simulink model "q3fullcontrolledSON"  (R2018a)
settings: Solver=VariableStepAuto  StartTime=0.0  StopTime=2  RelTol=1e-6
libraries: powerlib x14, powerlib_meascontrol x2
settings Model: Creator=asus  LastModifiedBy=asus

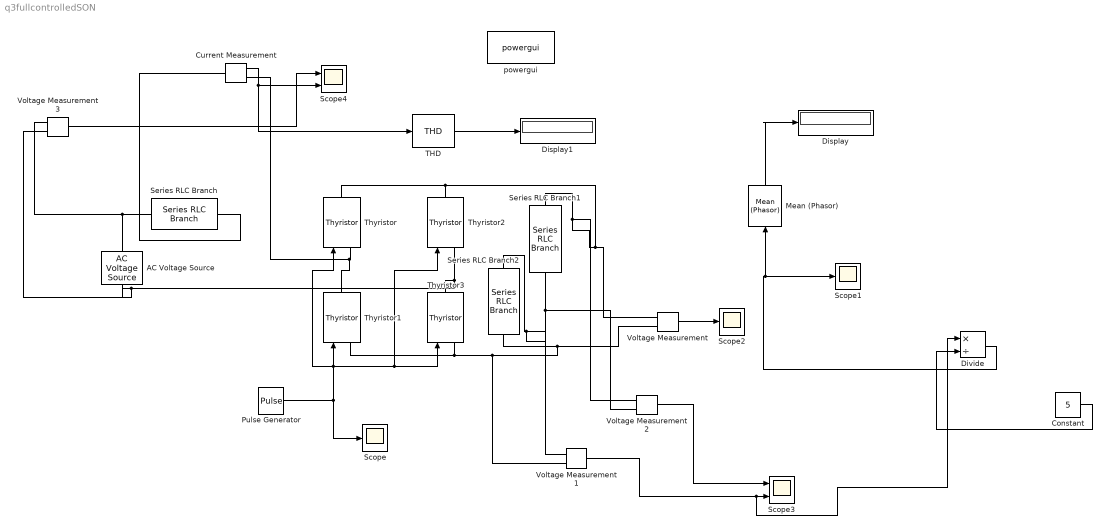
== system q3fullcontrolledSON ==
  AC Voltage Source : powerlib/Electrical Sources/AC Voltage Source  Amplitude=325.2  Phase=0  Frequency=50  SampleTime=0  Measurements=None  BusType=swing  Pref=10e3  Qref=0  Qmin=-inf  Qmax=+inf
  Constant : Constant  Value=5
  Current Measurement : powerlib/Measurements/Current Measurement  PhasorSimulation=off  OutputType=Complex  PSBequivalent=0
  Display : Display
  Display1 : Display
  Divide : Product  Inputs=*/
  Mean (Phasor) : powerlib_meascontrol/Measurements/Mean (Phasor)  Freq=60  Vinit=0  Ts=0
      settings: SourceProductName=Simscape Power Systems  SourceProductBaseCode=PS
  Pulse Generator : DiscretePulseGenerator  PulseType=Time based  Amplitude=10  Period=1e-2  PulseWidth=5  PhaseDelay=2.41e-3
  Scope : Scope
  Scope1 : Scope
  Scope2 : Scope
  Scope3 : Scope  NumInputPorts=2
  Scope4 : Scope  NumInputPorts=2
  Series RLC Branch : powerlib/Elements/Series RLC Branch  LConnTagsString=__new0  RConnTagsString=__new0  BranchType=L  Resistance=1  Inductance=5e-4  SetiL0=off  InitialCurrent=0  Capacitance=1e-6  Setx0=off  InitialVoltage=0  Measurements=None
  Series RLC Branch1 : powerlib/Elements/Series RLC Branch  LConnTagsString=__new0  RConnTagsString=__new0  BranchType=L  Resistance=1  Inductance=250e-3  SetiL0=off  InitialCurrent=0  Capacitance=1e-6  Setx0=off  InitialVoltage=0  Measurements=None
  Series RLC Branch2 : powerlib/Elements/Series RLC Branch  LConnTagsString=__new0  RConnTagsString=__new0  BranchType=R  Resistance=5  Inductance=1e-3  SetiL0=off  InitialCurrent=0  Capacitance=1e-6  Setx0=off  InitialVoltage=0  Measurements=None
  THD : powerlib_meascontrol/Measurements/THD  Freq=60  Ts=0
  Thyristor{,1..3} (4 alike) : powerlib/Power Electronics/Thyristor  Ron=1e-9  Lon=0  Vf=0  IC=0  Rs=500  Cs=1e-9  Measurements=off
  Voltage Measurement{,1..3} (4 alike) : powerlib/Measurements/Voltage Measurement  PhasorSimulation=off  OutputType=Complex  PSBequivalent=0
  powergui : powerlib/powergui  Priority=1  SimulationMode=Discrete  SampleTime=5e-6  frequency=60  Iterations=50  frequencyindice=50  Pbase=100e6  ErrMax=1e-4  UnitsV=kV  UnitsW=MW  buscounter=0  FunctionMessages=off  echomessages=off  EnableUseOfTLC=off  CurrentSourceSwitches=off  DisableSnubberDevices=off  DisableRonSwitches=off  DisableVfSwitches=off  DisplayEquations=off  SolverType=Tustin/Backward Euler (TBE)  Interpol=off  ExternalGateDelay=off  methode=off  Ts=100  x0status=blocks  SPID=on  SwTol=0  HookPort=off  RestoreLinks=warning  ResistiveCurrentMeasurement=off  Frange=[0:2:500]  Ylog=off  Xlog=on  ShowGrid=off  save=off  variable=ZData  structure=0  ZoomFFT=off  StartTime=0.0  cycles=1  DisplayStyle=1  fundamental=60  FreqAxis=off  MaxFrequency=1000  frequencyindicesteady=1  RmsSteady=1  display=off
  wires:
  Pulse Generator/1 -> Scope/1, Thyristor3/1, Thyristor2/1, Thyristor1/1, Thyristor/1
  Voltage Measurement/1 -> Scope2/1
  Voltage Measurement2/1 -> Scope3/1
  Voltage Measurement1/1 -> Divide/1, Scope3/2
  Constant/1 -> Divide/2
  Divide/1 -> Scope1/1, Mean (Phasor)/1
  Mean (Phasor)/1 -> Display/1
  Current Measurement/1 -> THD/1, Scope4/2
  Voltage Measurement3/1 -> Scope4/1
  THD/1 -> Display1/1
  connections:
  Series RLC Branch/LConn1 -- Voltage Measurement3/LConn1 -- AC Voltage Source/RConn1
  Current Measurement/LConn1 -- Series RLC Branch/RConn1
  Thyristor2/LConn1 -- Voltage Measurement3/LConn2 -- AC Voltage Source/LConn1 -- Thyristor3/RConn1
  Thyristor1/LConn1 -- Voltage Measurement1/LConn2 -- Voltage Measurement/LConn2 -- Series RLC Branch2/RConn1 -- Thyristor3/LConn1
  Thyristor/RConn1 -- Voltage Measurement2/LConn1 -- Series RLC Branch1/LConn1 -- Voltage Measurement/LConn1 -- Thyristor2/RConn1
  Series RLC Branch1/RConn1 -- Voltage Measurement2/LConn2 -- Voltage Measurement1/LConn1 -- Series RLC Branch2/LConn1
  Thyristor/LConn1 -- Current Measurement/RConn1 -- Thyristor1/RConn1
